simulink subsystem "senalizacion"  (R2024b)
settings: Solver=VariableStepAuto  StartTime=0.0  StopTime=10.0  RelTol=1e-3
settings Model: Creator=Usuario_UMA
settings RTWCC: GPUComputeCapability=3.5

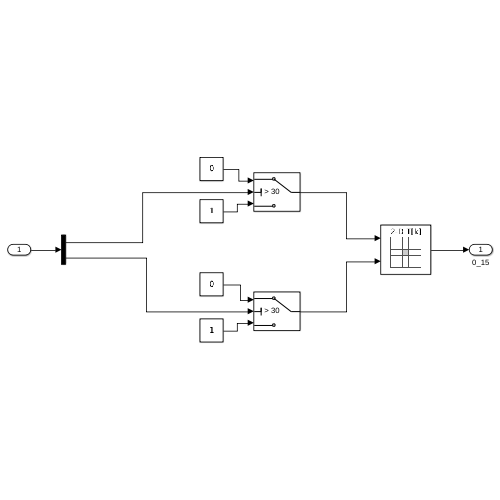
[thumbnail: Simulink's stored preview of the top-level diagram]
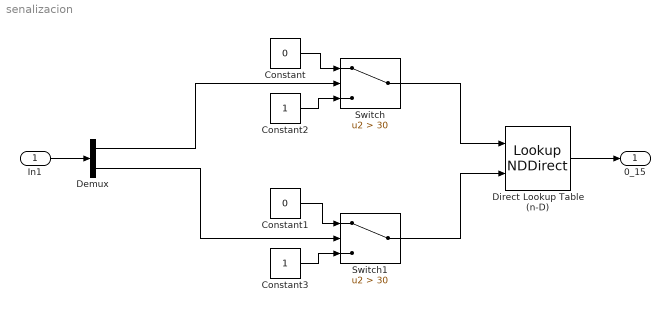
== system senalizacion ==
  In1 : Inport
  Constant : Constant  Value=0
  Constant1 : Constant  Value=0
  Constant2 : Constant
  Constant3 : Constant
  Demux : Demux  Outputs=2
  Direct Lookup Table (n-D) : LookupNDDirect  Table=[2 4;1 9]
  Switch : Switch  Criteria=u2 > Threshold  Threshold=30  SaturateOnIntegerOverflow=off  InputSameDT=off
  Switch1 : Switch  Criteria=u2 > Threshold  Threshold=30  SaturateOnIntegerOverflow=off  InputSameDT=off
  0_15 : Outport
  wires:
  In1/1 -> Demux/1
  Demux/1 -> Switch/2
  Constant/1 -> Switch/1
  Constant2/1 -> Switch/3
  Demux/2 -> Switch1/2
  Constant1/1 -> Switch1/1
  Constant3/1 -> Switch1/3
  Switch/1 -> Direct Lookup Table (n-D)/1
  Switch1/1 -> Direct Lookup Table (n-D)/2
  Direct Lookup Table (n-D)/1 -> 0_15/1
